simulink model "Vconc"  (R2023a)
settings: Solver=VariableStepAuto  StartTime=0.0  StopTime=10.0  RelTol=1e-3
undefined symbols (not defined in the file): C, K
settings Model: Creator=meghn  LastModifiedBy=meghn

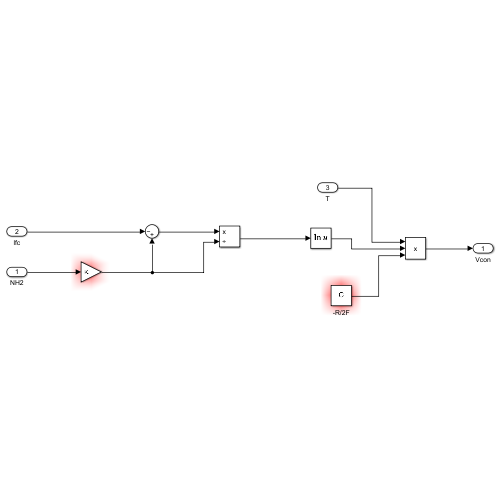
[thumbnail: Simulink's stored preview of the top-level diagram]
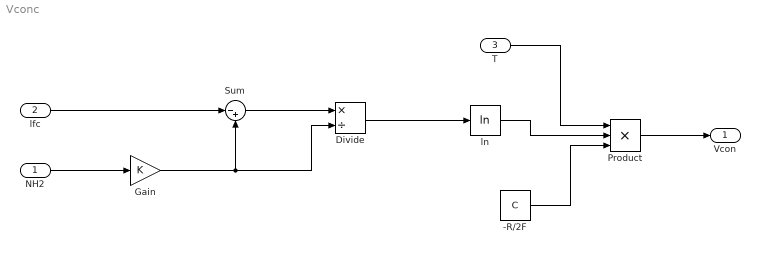
== system Vconc ==
  NH2 : Inport
  lfc : Inport  Port=2
  T : Inport  Port=3
  -R/2F : Constant  Value=C
  Divide : Product  Inputs=*/
  Gain : Gain  Gain=K
  Product : Product  Inputs=3
  Sum : Sum  Inputs=|-+
  ln : Math  Operator=log
  Vcon : Outport
  wires:
  NH2/1 -> Gain/1
  lfc/1 -> Sum/1
  Gain/1 -> Divide/2, Sum/2
  Sum/1 -> Divide/1
  Divide/1 -> ln/1
  T/1 -> Product/1
  ln/1 -> Product/2
  -R/2F/1 -> Product/3
  Product/1 -> Vcon/1
